simulink model "autonomyPipeline"  (R2026a)
settings: Solver=FixedStepAuto  StopTime=60  FixedStep=0.1
settings Model: Creator=ADITYA  LastModifiedBy=ADITYA

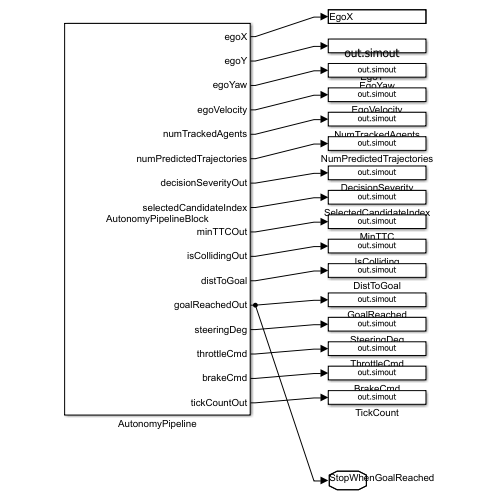
[thumbnail: Simulink's stored preview of the top-level diagram]
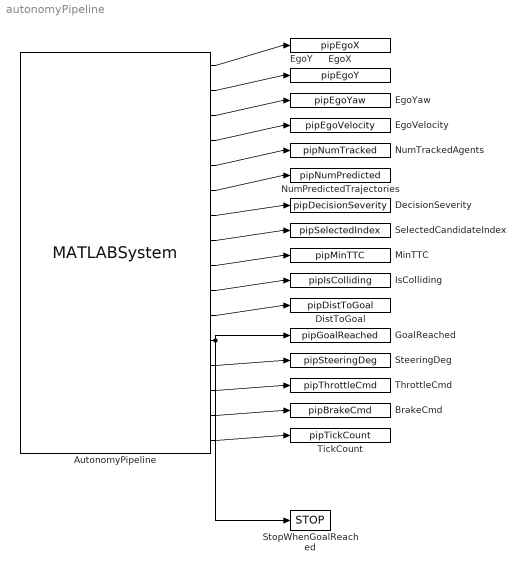
== system autonomyPipeline ==
  AutonomyPipeline : MATLABSystem  System=AutonomyPipelineBlock  ScenarioName=villageRoad  SimulateUsing=Interpreted execution
      mask Type: AutonomyPipelineBlock
  BrakeCmd : ToWorkspace  VariableName=pipBrakeCmd  SampleTime=-1
  DecisionSeverity : ToWorkspace  VariableName=pipDecisionSeverity  SampleTime=-1
  DistToGoal : ToWorkspace  VariableName=pipDistToGoal  SampleTime=-1
  EgoVelocity : ToWorkspace  VariableName=pipEgoVelocity  SampleTime=-1
  EgoX : ToWorkspace  VariableName=pipEgoX  SampleTime=-1
  EgoY : ToWorkspace  VariableName=pipEgoY  SampleTime=-1
  EgoYaw : ToWorkspace  VariableName=pipEgoYaw  SampleTime=-1
  GoalReached : ToWorkspace  VariableName=pipGoalReached  SampleTime=-1
  IsColliding : ToWorkspace  VariableName=pipIsColliding  SampleTime=-1
  MinTTC : ToWorkspace  VariableName=pipMinTTC  SampleTime=-1
  NumPredictedTrajectories : ToWorkspace  VariableName=pipNumPredicted  SampleTime=-1
  NumTrackedAgents : ToWorkspace  VariableName=pipNumTracked  SampleTime=-1
  SelectedCandidateIndex : ToWorkspace  VariableName=pipSelectedIndex  SampleTime=-1
  SteeringDeg : ToWorkspace  VariableName=pipSteeringDeg  SampleTime=-1
  StopWhenGoalReached : Stop
  ThrottleCmd : ToWorkspace  VariableName=pipThrottleCmd  SampleTime=-1
  TickCount : ToWorkspace  VariableName=pipTickCount  SampleTime=-1
  wires:
  AutonomyPipeline/1 -> EgoX/1
  AutonomyPipeline/2 -> EgoY/1
  AutonomyPipeline/3 -> EgoYaw/1
  AutonomyPipeline/4 -> EgoVelocity/1
  AutonomyPipeline/5 -> NumTrackedAgents/1
  AutonomyPipeline/6 -> NumPredictedTrajectories/1
  AutonomyPipeline/7 -> DecisionSeverity/1
  AutonomyPipeline/8 -> SelectedCandidateIndex/1
  AutonomyPipeline/9 -> MinTTC/1
  AutonomyPipeline/10 -> IsColliding/1
  AutonomyPipeline/11 -> DistToGoal/1
  AutonomyPipeline/12 -> GoalReached/1, StopWhenGoalReached/1
  AutonomyPipeline/13 -> SteeringDeg/1
  AutonomyPipeline/14 -> ThrottleCmd/1
  AutonomyPipeline/15 -> BrakeCmd/1
  AutonomyPipeline/16 -> TickCount/1
